simulink library "UsefulBlocksLibrary"  (R2014b)
settings: Solver=ode45  SolverMode=SingleTasking  StartTime=0.0  StopTime=10.0  RelTol=1e-3
undefined symbols (not defined in the file): ActuatorStruct, CalibrationAngles, drivePeakCurrent, JointAbsoluteEncoderCounts_rev, JointPositionGuardMax_rad, JointPositionGuardMin_rad, MotorEncoderCounts_rev, motorTorqueConstant, sampleTime, transmissionRatio
libraries: simulink x13, FM_Library x4, dspsigops x1, simulink_extras x1
(part 2 of 2)

== matlab function UsefulBlocksLibrary/FromActuator/DecodeEncoder ==
  data: Encoder_counts input; EncoderCounts_rev parameter; EncoderPosition_rad output
function EncoderPosition_rad = ...
    DecodeEncoder(Encoder_counts, EncoderCounts_rev)
%#codegen

% This block decodes the motor encoder counts to the motor angle

EncoderPosition_rad = (double(Encoder_counts) / EncoderCounts_rev * 2 * pi);

== matlab function UsefulBlocksLibrary/FromActuator/DecodeEncoder1 ==
  data: Encoder_counts input; EncoderCounts_rev parameter; EncoderPosition_rad output
function EncoderPosition_rad = ...
    DecodeEncoder(Encoder_counts, EncoderCounts_rev)
%#codegen

% This block decodes the motor encoder counts to the motor angle

EncoderPosition_rad = (double(Encoder_counts) / EncoderCounts_rev * 2 * pi);

== matlab function UsefulBlocksLibrary/ToActuator/DriveEnableLogic/enableDrive (CoE) ==
  data: ControlWord output; enable input; TimePerState_ms input
function ControlWord = enabledrive(enable, TimePerState_ms)
%#codegen
%
% Input arguments:
% enable:
%   0: Disable drive
%   Any non-zero: enable drive.
% TimePerState_ms:
%   A four-element array containing the time in ms for each state (states
%   are: 0, 128, 6, 7. The final state, 15, is kept until drive needs to be
%   disabled again.
%
% Changing enable forces the initialize-sequence to run
persistent previousEnable;
persistent counter;
if isempty(previousEnable)
    previousEnable = enable; % No enabling of the drive at startup
    counter = 1e6;
end;

if enable~=previousEnable
    counter = 0;
end;
previousEnable = enable;

TimePerState_cum = cumsum(TimePerState_ms);

if enable~=0
    counter = counter+1;
    if counter < TimePerState_cum(1);
        ControlWord_ = 0;
    elseif counter < TimePerState_cum(2);
        ControlWord_ = 128;
    elseif counter < TimePerState_cum(3);
        ControlWord_ = 6;
    elseif counter < TimePerState_cum(4);
        ControlWord_ = 7;
    else
        ControlWord_ = 15;
    end
else
    ControlWord_ = 6;
end

ControlWord = uint16(ControlWord_);

== matlab function UsefulBlocksLibrary/FromActuator/CalibrateMotorPosition     ==
  data: MotorPosition_rad input; MotorPositionCalibrated_rad output; JointPosition_IncEnc_rad output; transmissionRatio parameter; JointPosition_AbsEnc_rad input; Calibrate input; CalibrationAngle input
function [MotorPositionCalibrated_rad, JointPosition_IncEnc_rad]...
    = CalibrateMotorPosition( MotorPosition_rad, transmissionRatio, JointPosition_AbsEnc_rad, Calibrate, CalibrationAngle)
%#codegen

% This block includes calibration such that (ideally) the motor angle is
% zero when the joint angle and spring deflection are zero as well. Before
% the calibration has occurred, the output of this function is -1e9*. This
% is chosen such that the value is always outside the allowed motor angle
% range; this prevents the drive from being allowed to turn on.
% 
% * I wanted to use -inf as starting function, but I'm not sure whether
%   that will be handled correctly in all cases.

persistent isCalibrated;
persistent offset;

if isempty(isCalibrated) % no calibration needed
    isCalibrated = 1;
    offset = 0;
end;


if Calibrate
%     if ~isempty(JointPosition_AbsEnc_rad)
%         target_pos_mot_rad = transmissionRatio * JointPosition_AbsEnc_rad; % This is what we should read
        target_pos_mot_rad = CalibrationAngle; % This is what we should read / fix for now
        offset = target_pos_mot_rad*transmissionRatio - MotorPosition_rad; % calculate offset
%     else
%         % no absolute encoder data available, offset is zero
%         offset = 0;
%     end
    isCalibrated = 1;
end;

% if already calibrated, calculate calibrated motor angle
if isCalibrated
    MotorPositionCalibrated_rad = MotorPosition_rad + offset;
    JointPosition_IncEnc_rad = MotorPositionCalibrated_rad / transmissionRatio;
else
    MotorPositionCalibrated_rad = MotorPosition_rad;
    JointPosition_IncEnc_rad = MotorPositionCalibrated_rad / transmissionRatio;
end;

== matlab function UsefulBlocksLibrary/EndstopAndSafety/MATLAB Function ==
  data: deltaX input; v_limit output; MaxAcc input; ReturnVelocity input; ReturnVelocitySlope input
function v_limit = fcn(deltaX, MaxAcc, ReturnVelocity,ReturnVelocitySlope)
% Note: all input parameters should be positive!
% deltaX should be positive while in the 'allowed' region. If needed,
% negate the input to get it such.
%
% For the output: the v_limit is positive when in the 'allowed' region. if
% needed, negate the output to get it such.

%#codegen

if deltaX>=0
    v_limit = sqrt(2*MaxAcc * deltaX);
else
    v_limit = max ([deltaX*ReturnVelocitySlope, -ReturnVelocity]); 
end;

== matlab function UsefulBlocksLibrary/EndstopAndSafety/MATLAB Function1 ==
  data: deltaX input; v_limit output; MaxAcc input; ReturnVelocity input; ReturnVelocitySlope input
function v_limit = fcn(deltaX, MaxAcc, ReturnVelocity,ReturnVelocitySlope)
% Note: all input parameters should be positive!
% deltaX should be positive while in the 'allowed' region. If needed,
% negate the input to get it such.
%
% For the output: the v_limit is positive when in the 'allowed' region. if
% needed, negate the output to get it such.

%#codegen

if deltaX>=0
    v_limit = sqrt(2*MaxAcc * deltaX);
else
    v_limit = max ([deltaX*ReturnVelocitySlope, -ReturnVelocity]); 
end;

== matlab function UsefulBlocksLibrary/FromActuator/CheckOperationEnabled ==
  data: u input; y output
function y = fcn(u)
%#codegen

mask  = bin2dec('0000000001101111');
match = bin2dec('0000000000100111');

masked = bitand(u,mask);
if masked==match
    y=1;
else
    y=0;
end;

== matlab function UsefulBlocksLibrary/DecodeEncoder ==
  data: Encoder_counts input; EncoderCounts_rev parameter; EncoderPosition_rad output
function EncoderPosition_rad = ...
    DecodeEncoder(Encoder_counts, EncoderCounts_rev)
%#codegen

% This block decodes the motor encoder counts to the motor angle

EncoderPosition_rad = (double(Encoder_counts) / EncoderCounts_rev * 2 * pi);

== matlab function UsefulBlocksLibrary/ToActuator/EncodeDesiredTorque ==
  data: MotorTorque_Des_IU output int16; JointTorque_Des_Nm input; transmissionRatio parameter; motorTorqueConstant parameter; drivePeakCurrent parameter
function MotorTorque_Des_IU = EncodeDesiredTorque(JointTorque_Des_Nm, transmissionRatio, motorTorqueConstant, drivePeakCurrent)
%#codegen
% Calculate the target torque in incremental units for a desired joint
% torque.

% compute torque at motor (negate because sign change due to transmission)
torque_motor = JointTorque_Des_Nm / transmissionRatio; 

% desired current (i_des) = torque_motor / kt (torque constant)
i_des = torque_motor / motorTorqueConstant;

% calculate the target torque in incremental units [IU], see CoE manual
% Technosoftmotion
MotorTorque_Des_IU = int16( 65520*i_des / (2*drivePeakCurrent) );

== matlab function UsefulBlocksLibrary/ToActuator/DriveEnableLogic/CreateSingleErrorValue/MATLAB Function ==
  data: errors input; out output
function out = errorToPowerOf2(errors)
%#codegen

% if size(errors,1) > size(errors,2)
%     errors = errors.';
% end
out = sum(errors.*(2.^(0:(length(errors)-1)).'));

== matlab function UsefulBlocksLibrary/SmoothTransition/Subsystem/MATLAB Function ==
  data: t input; smooth output; Ttransition parameter
function smooth = smootherstep(t,Ttransition )
%#codegen
% smootherstep, based on Perlin
% 1st and 2nd derivatives are 0 at edges

if (t <= Ttransition)
    smooth = (t/Ttransition).^3 .* (6*(t/Ttransition).^2 -15*(t/Ttransition) +10);
else
    smooth = 1;
end
